simulink model "buck"  (R2015a)
settings: Solver=ode3  StartTime=0  StopTime=Tend  FixedStep=1e-5  RelTol=1e-3
InitFcn:
  | BatteryModel
  | EV_bidirectional_boost_parameters
values from neighbouring files (symbols this model uses):
  Co = 1186.5e-6    (= 0.0011865)    [config.m]
  Fc = 2000    [config.m]
  Imax = 250    [config.m]
  Kii = 5*R/L    (= 50)    [config.m]
  Kiv = 5    [config.m]
  Kpi = 2*pi*bw*L*5    (= 1099.55742876)    [config.m]
  Kpv = 2*pi*bwv*Co    (= 0.223649981009)    [config.m]
  L = 50e-3    (= 0.05)    [config.m]
  R = 0.5    [config.m]
  Tstart = 0.5    [config.m]
  VLmax = VBNmax    [config.m]
  Vo_ref = 565    [config.m]
undefined symbols (not defined in the file or in its folder): Ion, Lithium
libraries: powerlib x11, simulink x5, electricdrivelib x1
settings Model: Creator=Mert Karadeniz  LastModifiedBy=MERT KARADENIZ
settings DebuggingCC: UnderspecifiedInitializationDetection=Classic  MergeDetectMultiDrivingBlocksExec=none  SolverPrmCheckMsg=warning  StateNameClashWarn=warning

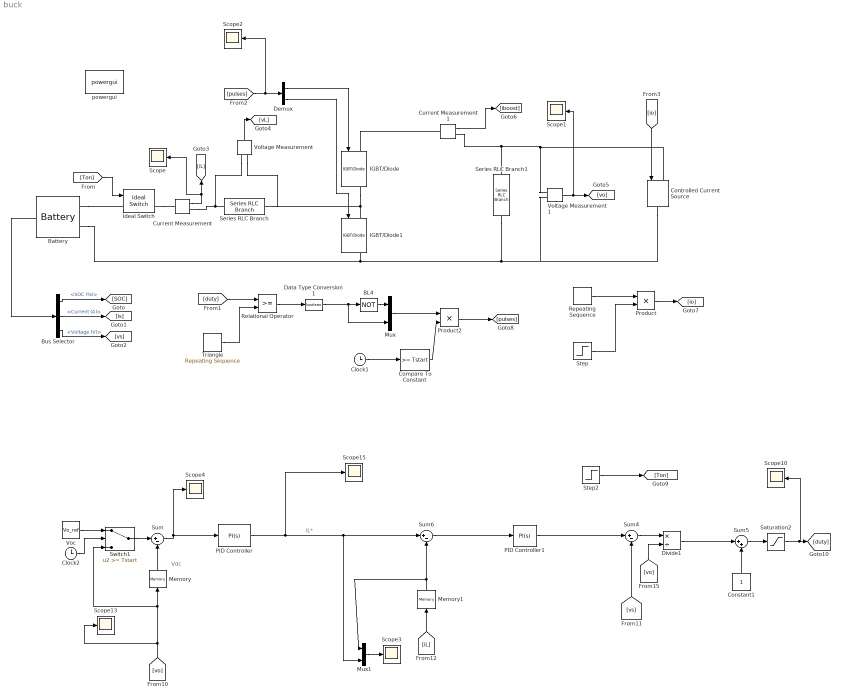
== system buck ==
  note: iL*
  note: Vdc
  BL4 : Logic  Operator=NOT  Inputs=1
  Battery : electricdrivelib/Extra Sources/Battery  BatType=Lithium-Ion  ShowDetailedParameters=off  NomV=VBN  NomQ=RC  SOC=SOCo  PresetModel=on  MaxQ=66.6667  FullV=419.0354  Dis_rate=28.9855  R=0.054  Normal_OP=60.2899  expZone="[388.9389      3.275362]"  current=[1.5 3]  Units=Ampere-hour  Batt_Tr=BATRESPONSETIME
  Bus Selector : BusSelector  OutputSignals=SOC (%),Current (A),Voltage (V)
  Clock1 : Clock
  Clock2 : Clock
  Compare To Constant : simulink/Logic and Bit Operations/Compare To Constant  relop=>=  const=Tstart  OutDataTypeStr=boolean
  Constant1 : Constant
  Controlled Current Source : powerlib/Electrical Sources/Controlled Current Source  Initialize=on  Source_Type=AC  Amplitude=0  Phase=0  Frequency=0  Measurements=None
  Current Measurement : powerlib/Measurements/Current Measurement  PhasorSimulation=off  OutputType=Complex  PSBequivalent=0
  Current Measurement1 : powerlib/Measurements/Current Measurement  PhasorSimulation=off  OutputType=Complex  PSBequivalent=0
  Data Type Conversion1 : DataTypeConversion  OutDataTypeStr=boolean  SaturateOnIntegerOverflow=on  RndMeth=Zero
  Demux : Demux  Outputs=2
  Divide1 : Product  Inputs=*/
  IGBT/Diode : powerlib/Power Electronics/IGBT//Diode  Ron=1e-3  Rs=1e5  Cs=inf  Measurements=on
  IGBT/Diode1 : powerlib/Power Electronics/IGBT//Diode  Ron=1e-3  Rs=1e5  Cs=inf  Measurements=on
  Ideal Switch : powerlib/Power Electronics/Ideal Switch  Ron=0.001  Lon=0  IC=0  Rs=1e5  Cs=inf  Measurements=on
  Memory : Memory  InheritSampleTime=on  LinearizeAsDelay=on
  Memory1 : Memory  InheritSampleTime=on  LinearizeAsDelay=on
  Mux : Mux  Inputs=2
  Mux1 : Mux  Inputs=2
  PID Controller : simulink/Continuous/PID Controller  Controller=PI  TimeDomain=Continuous-time  SampleTime=-1  IntegratorMethod=Forward Euler  FilterMethod=Forward Euler  Form=Ideal  UseFilter=on  ControllerParametersSource=internal  P=Kpv  I=Kiv  D=0  N=100  InitialConditionSource=internal  InitialConditionForIntegrator=0  InitialConditionForFilter=0  ExternalReset=none  LimitOutput=on  UpperSaturationLimit=Imax  LowerSaturationLimit=-Imax  LinearizeAsGain=on  AntiWindupMode=back-calculation  Kb=10  TrackingMode=off  Kt=1  PParamMin=[]  PParamMax=[]  IParamMin=[]  IParamMax=[]  DParamMin=[]  DParamMax=[]  NParamMin=[]  NParamMax=[]  KbParamMin=[]  KbParamMax=[]  KtParamMin=[]  KtParamMax=[]  POutMin=[]  POutMax=[]  IOutMin=[]  IOutMax=[]  DOutMin=[]  DOutMax=[]  NOutMin=[]  NOutMax=[]  KbOutMin=[]  KbOutMax=[]  KtOutMin=[]  KtOutMax=[]  IntegratorOutMin=[]  IntegratorOutMax=[]  FilterOutMin=[]  FilterOutMax=[]  SumOutMin=[]  SumOutMax=[]  SumI1OutMin=[]  SumI1OutMax=[]  SumI2OutMin=[]  SumI2OutMax=[]  SumI3OutMin=[]  SumI3OutMax=[]  SumDOutMin=[]  SumDOutMax=[]  SaturationOutMin=[]  SaturationOutMax=[]  IntegratorContinuousStateAttributes=''  IntegratorStateMustResolveToSignalObject=off  IntegratorRTWStateStorageClass=Auto  FilterContinuousStateAttributes=''  FilterStateMustResolveToSignalObject=off  FilterRTWStateStorageClass=Auto  DifferentiatorICPrevScaledInput=0  DifferentiatorOutMin=[]  DifferentiatorOutMax=[]
  PID Controller1 : simulink/Continuous/PID Controller  Controller=PI  TimeDomain=Continuous-time  SampleTime=-1  IntegratorMethod=Forward Euler  FilterMethod=Forward Euler  Form=Ideal  UseFilter=on  ControllerParametersSource=internal  P=Kpi  I=Kii  D=0  N=100  InitialConditionSource=internal  InitialConditionForIntegrator=0  InitialConditionForFilter=0  ExternalReset=none  LimitOutput=on  UpperSaturationLimit=VLmax  LowerSaturationLimit=-VLmax  LinearizeAsGain=on  AntiWindupMode=clamping  Kb=1  TrackingMode=off  Kt=1  PParamMin=[]  PParamMax=[]  IParamMin=[]  IParamMax=[]  DParamMin=[]  DParamMax=[]  NParamMin=[]  NParamMax=[]  KbParamMin=[]  KbParamMax=[]  KtParamMin=[]  KtParamMax=[]  POutMin=[]  POutMax=[]  IOutMin=[]  IOutMax=[]  DOutMin=[]  DOutMax=[]  NOutMin=[]  NOutMax=[]  KbOutMin=[]  KbOutMax=[]  KtOutMin=[]  KtOutMax=[]  IntegratorOutMin=[]  IntegratorOutMax=[]  FilterOutMin=[]  FilterOutMax=[]  SumOutMin=[]  SumOutMax=[]  SumI1OutMin=[]  SumI1OutMax=[]  SumI2OutMin=[]  SumI2OutMax=[]  SumI3OutMin=[]  SumI3OutMax=[]  SumDOutMin=[]  SumDOutMax=[]  SaturationOutMin=[]  SaturationOutMax=[]  IntegratorContinuousStateAttributes=''  IntegratorStateMustResolveToSignalObject=off  IntegratorRTWStateStorageClass=Auto  FilterContinuousStateAttributes=''  FilterStateMustResolveToSignalObject=off  FilterRTWStateStorageClass=Auto  DifferentiatorICPrevScaledInput=0  DifferentiatorOutMin=[]  DifferentiatorOutMax=[]
  Product : Product
  Product2 : Product  RndMeth=Zero
  Relational Operator : RelationalOperator
  Repeating Sequence : simulink/Sources/Repeating Sequence  rep_seq_t=[0 2 4 6 8]  rep_seq_y=[0 2 0 -2 0]*5
  Saturation2 : Saturate  UpperLimit=1  LowerLimit=0
  Scope{,1..4,10,13,15} (8 alike) : Scope
      Scope settings: YMin=0.00389075  YMax=0.00389475
      Scope1 settings: YMin=400  YMax=775
      Scope10 settings: TimeRange=8  YMin=0.95  YMax=1.05  SaveName=ScopeData2
      Scope13 settings: TimeRange=8  YMin=11.725  YMax=11.975  SaveName=ScopeData3
      Scope15 settings: TimeRange=8  YMin=250  YMax=250  SaveName=ScopeData4
      Scope2 settings: TimeRange=8  YMin=0.95  YMax=1.05  SaveName=ScopeData5
      Scope3 settings: TickLabels=on  TimeRange=8  YMin=-70  YMax=60  SaveName=ScopeData6
      Scope4 settings: TimeRange=8  YMin=0  YMax=600  SaveName=ScopeData7
  Series RLC Branch : powerlib/Elements/Series RLC Branch  LConnTagsString=__new0  RConnTagsString=__new0  BranchType=RL  Resistance=R  Inductance=L  SetiL0=off  InitialCurrent=0  Capacitance=1e-6  Setx0=off  InitialVoltage=0  Measurements=None
  Series RLC Branch1 : powerlib/Elements/Series RLC Branch  LConnTagsString=__new0  RConnTagsString=__new0  BranchType=C  Resistance=1  Inductance=1e-3  SetiL0=off  InitialCurrent=0  Capacitance=Co  Setx0=on  InitialVoltage=Vs_full  Measurements=Branch voltage and current
  Step : Step  Time=1.5  SampleTime=0
  Step2 : Step  Time=Tstart  SampleTime=0
  Sum : Sum  Inputs=|+-
  Sum4 : Sum  Inputs=|+-
  Sum5 : Sum  Inputs=|++
  Sum6 : Sum  Inputs=|+-
  Switch1 : Switch  Threshold=Tstart
  Triangle : simulink/Sources/Repeating Sequence  rep_seq_t=[0 1/Fc/2 1/Fc]  rep_seq_y=[0 1 0]
  Voc : Constant  Value=Vo_ref
  Voltage Measurement : powerlib/Measurements/Voltage Measurement  PhasorSimulation=off  OutputType=Complex  PSBequivalent=0
  Voltage Measurement1 : powerlib/Measurements/Voltage Measurement  PhasorSimulation=off  OutputType=Complex  PSBequivalent=0
  powergui : powerlib/powergui  Priority=1  SimulationMode=Discrete  SolverType=Tustin  SampleTime=10e-6  frequency=60  SPID=off  DisableSnubberDevices=off  DisableRonSwitches=off  DisableVfSwitches=off  SwTol=0  DisplayEquations=off  Interpol=off  methode=off  Ts=0  FunctionMessages=off  echomessages=off  HookPort=off  EnableUseOfTLC=off  x0status=blocks  frequencyindice=0  Pbase=100e6  ErrMax=1e-4  Iterations=50  UnitsV=kV  UnitsW=MW  buscounter=0  RestoreLinks=warning  ResistiveCurrentMeasurement=off  Frange=[0:2:500]  Ylog=off  Xlog=on  ShowGrid=off  save=off  variable=ZData  structure=0  ZoomFFT=off  StartTime=0.0  cycles=1  DisplayStyle=1  fundamental=60  FreqAxis=off  MaxFrequency=1000  frequencyindicesteady=1  RmsSteady=1  display=off
  wires:
  Battery/1 -> Bus Selector/1
  Bus Selector/1 -> [SOC]  "<SOC (%)>"
  Bus Selector/2 -> [is]  "<Current (A)>"
  Bus Selector/3 -> [vs]  "<Voltage (V)>"
  Demux/1 -> IGBT/Diode/1
  Demux/2 -> IGBT/Diode1/1
  Voltage Measurement/1 -> [vL]
  Current Measurement/1 -> Scope/1, [iL]
  [Ton] -> Ideal Switch/1
  Voltage Measurement1/1 -> Scope1/1, [vo]
  Current Measurement1/1 -> [iboost]
  Repeating Sequence/1 -> Product/1
  Step/1 -> Product/2
  Product/1 -> [io]
  Relational Operator/1 -> Data Type Conversion1/1
  [duty] -> Relational Operator/1
  Triangle/1 -> Relational Operator/2
  Data Type Conversion1/1 -> Mux/2, BL4/1
  BL4/1 -> Mux/1
  Mux/1 -> Product2/1
  Clock1/1 -> Compare To Constant/1
  Compare To Constant/1 -> Product2/2
  Product2/1 -> [pulses]
  [pulses] -> Scope2/1, Demux/1
  [vs] -> Sum4/2
  Sum4/1 -> Divide1/1
  [vo] -> Divide1/2
  Divide1/1 -> Sum5/1
  Constant1/1 -> Sum5/2
  Sum5/1 -> Saturation2/1
  [vo] -> Memory/1, Switch1/3, Scope13/1
  Clock2/1 -> Switch1/2
  Voc/1 -> Switch1/1
  Switch1/1 -> Sum/1
  PID Controller/1 -> Mux1/2, Sum6/1, Scope15/1
  PID Controller1/1 -> Sum4/1
  Saturation2/1 -> Scope10/1, [duty]
  [io] -> Controlled Current Source/1
  Mux1/1 -> Scope3/1
  Step2/1 -> [Ton]
  Memory/1 -> Sum/2
  Sum/1 -> Scope4/1, PID Controller/1
  Sum6/1 -> PID Controller1/1
  [iL] -> Memory1/1
  Memory1/1 -> Mux1/1, Sum6/2
  connections:
  Battery/LConn1 -- Ideal Switch/LConn1
  IGBT/Diode/RConn1 -- Voltage Measurement/LConn2 -- Series RLC Branch/RConn1 -- IGBT/Diode1/LConn1
  IGBT/Diode/LConn1 -- Current Measurement1/LConn1
  Controlled Current Source/RConn1 -- Voltage Measurement1/LConn2 -- Series RLC Branch1/RConn1 -- Battery/LConn2 -- IGBT/Diode1/RConn1
  Ideal Switch/RConn1 -- Current Measurement/LConn1
  Current Measurement/RConn1 -- Voltage Measurement/LConn1 -- Series RLC Branch/LConn1
  Controlled Current Source/LConn1 -- Current Measurement1/RConn1 -- Series RLC Branch1/LConn1 -- Voltage Measurement1/LConn1
